simulink model "msePardoSplitOfTwo"  (R2024b)
settings: Solver=VariableStepAuto  StartTime=0.0  StopTime=10.0  RelTol=1e-3
settings Model: Creator=DarianMuresan  LastModifiedBy=ferbe
settings RTWCC: GPUComputeCapability=3.5

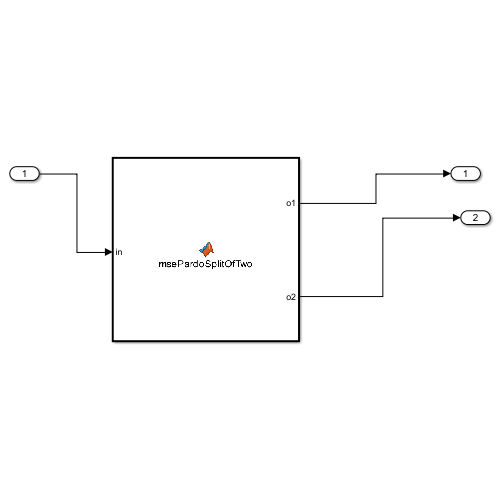
[thumbnail: Simulink's stored preview of the top-level diagram]
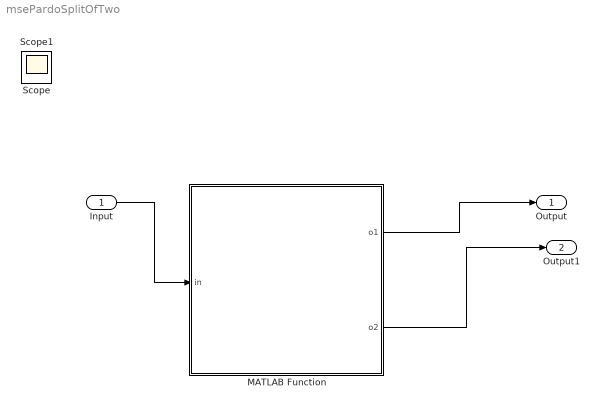
== system msePardoSplitOfTwo ==
  Input : Inport
  MATLAB Function : MATLAB Function  TreatAsAtomicUnit=on
  Output : Outport
  Output1 : Outport  Port=2
  Scope : Scope
  Scope1 : Scope
  wires:
  MATLAB Function/1(o1) -> Output/1
  MATLAB Function/2(o2) -> Output1/1
  Input/1 -> MATLAB Function/1(in)

== matlab function msePardoSplitOfTwo/MATLAB Function ==
  data: in input; o1 output; o2 output
function [o1,o2] = msePardoSplitOfTwo(in)

% Method to demux input into one of 4 possible outputs based on
% the assumption that processes run in parallel and they must all complete.
%
% A non-valid output is negative
%
% Written by: Darian Muresan
% Last Modified: 10/10/2024

if in<0
    o1 = -1;
    o2 = -1;
else
    o1 = in;
    o2 = in;  
end
